simulink model "D_20210914_Modell_Inbetriebnahme_BreakOutBox_Jetson"  (R2021a)
settings: Solver=ode1  StartTime=0.0  StopTime=500  FixedStep=Ts  RelTol=1e-3
PreLoadFcn:
  | pulsePeriod = 0.05;
  | 
  | Ts = 0.001;
  | 
  | FPGA_Frequency = 75000000;
  | 
  | ts_IO691 = 5e-3;
PostLoadFcn:
  | ewolfSetUp
InitFcn:
  | pulsePeriod = 0.05;
  | 
  | Ts = 0.001;
  | 
  | FPGA_Frequency = 75000000;
  | 
  | ts_IO691 = 5e-3;
StopFcn:
  | Simulink.sdi.clearPreferences;
  | if isfile(['sdi_view_',bdroot,'.mldatx'])
  | Simulink.sdi.view;
  | pause(3);
  | Simulink.sdi.loadView(['sdi_view_',bdroot,]);
  | end
values from neighbouring files (symbols this model uses):
  max_ac = 2    [ewolfSetUp.m]
  max_steer = 0.26    [ewolfSetUp.m]
  min_ac = -3    [ewolfSetUp.m]
  min_steer = -0.26    [ewolfSetUp.m]
  PredictionHorizon = 30    [ewolfSetUp.m]
undefined symbols (not defined in the file or in its folder): canChannel, DiscIntNeverNeededParam, Ended, HS, IO291, IO397, Single
libraries: lllalib x255, canmsglib x143, simulink x33, speedgoatlib_IO191 x5, speedgoatlib_IO291 x5, speedgoatlib_IO691 x3, slrealtimeiplib x2, simulink_extras x1, speedgoatlib_fpga_dio x1, speedgoatlib_fpga_quadrature x1, speedgoatlib_fpga x1, canlib x1
(part 7 of 7)

== system D_20210914_Modell_Inbetriebnahme_BreakOutBox_Jetson/IO691/CAN Read Loop - Port 3/Enabled Subsystem/extract radar data from CAN msg stream/Subsystem100/Subsystem9 ==
  reset : Inport
  data : Inport  Port=2
  saveBool : Inport  Port=3
  Mux : Mux  Inputs=10
  saveData{,1..9} (10 alike) : lllalib/saveData  SystemSampleTime=-1  VariantActivationTime=update diagram  Latency=0  AutoFrameSizeCalculation=off
  out : Outport
  nextSave : Outport  Port=2
  wires:
  saveData3/2 -> Mux/4
  saveData8/1 -> saveData9/2
  saveData7/1 -> saveData8/2
  reset/1 -> saveData/1, saveData1/1, saveData2/1, saveData3/1, saveData4/1, saveData5/1, saveData6/1, saveData8/1, saveData9/1, saveData7/1
  saveData3/1 -> saveData4/2
  saveData4/1 -> saveData5/2
  saveData2/2 -> Mux/3
  Mux/1 -> out/1
  saveData6/2 -> Mux/7
  saveData9/1 -> nextSave/1
  saveData4/2 -> Mux/5
  saveData5/1 -> saveData6/2
  saveData/2 -> Mux/1
  saveData8/2 -> Mux/9
  data/1 -> saveData/2
  saveData7/2 -> Mux/8
  saveData/1 -> saveData1/2
  saveData9/2 -> Mux/10
  saveData6/1 -> saveData7/2
  saveData2/1 -> saveData3/2
  saveData5/2 -> Mux/6
  saveData1/1 -> saveData2/2
  saveData1/2 -> Mux/2
  saveBool/1 -> saveData/3, saveData1/3, saveData2/3, saveData3/3, saveData4/3, saveData5/3, saveData6/3, saveData7/3, saveData8/3, saveData9/3

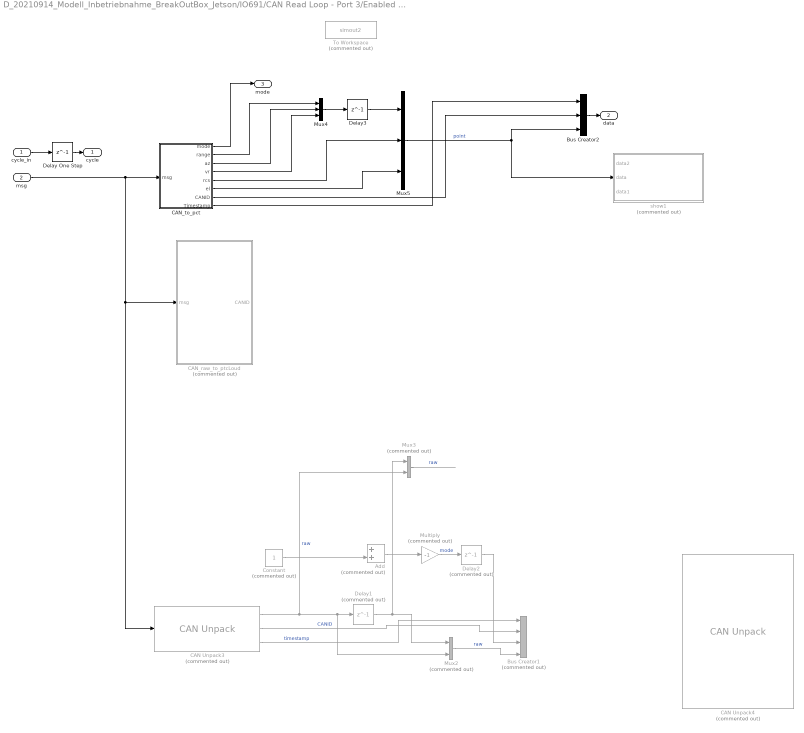
== system D_20210914_Modell_Inbetriebnahme_BreakOutBox_Jetson/IO691/CAN Read Loop - Port 3/Enabled Subsystem/extract radar data from CAN msg stream/extract point from CAN msg/extract radar_CAN_data (each cycle) ==
  cycle_in : Inport
  msg : Inport  Port=2
  Add : Sum  Commented=on
  Bus Creator1 : BusCreator  Commented=on  Inputs=4
  Bus Creator2 : BusCreator  Inputs=3
  CAN Unpack3 : canmsglib/CAN Unpack  Commented=on  MsgList=(none)  MsgName=CAN Msg  MsgIDType=Standard (11-bit identifier)  MsgIdentifier=-1  MsgLength=8  SignalInfo={}  IDPort=on  TimestampPort=on  ErrorPort=off  RemotePort=off  LengthPort=off  StatusPort=off  ApplyMinMax=off
      settings: SourceProductBaseCode=ME,XP,VN  DataFormat=raw data
  CAN Unpack4 : canmsglib/CAN Unpack  Commented=on  MsgList=(none)  MsgName=CAN Msg  MsgIDType=Standard (11-bit identifier)  MsgIdentifier=-1  MsgLength=8  SignalInfo={ 'Mode', '0', '1', 'LE', 'unsigned', 'Multiplexor', '0', '1', '0', '-Inf', 'Inf'; 'Range', '1', '13', 'LE', 'unsigned', 'Multiplexed', '0', '0.04', '0', '-Inf', 'Inf'; 'int1', '14', '8', 'LE', 'unsigned', 'Multiplexed', '0', '1', '0', '-Inf', 'Inf'; 'az', '22', '10', 'LE', 'unsigned', 'Multiplexed', '0', '1', '0', '-Inf', 'Inf'; 'int2', '32', '7', 'LE', 'unsigned', 'Multiplexed', '0', '1', '0', '-Inf', 'Inf'; 'vr', '39', '12', 'LE', 'unsigned', 'Multiplexed', '0', '0.04', '2992', '-44.12', '119.68'; 'int3', '51', '7', 'LE', 'unsigned', 'Multiplexed', '0', '1', '0', '-Inf', 'Inf'; 'int4', '58', '6', 'LE', 'unsigned', 'Multiplexed', '0', '1', '0', '-Inf', 'Inf'; 'rcs', '1', '8', 'LE', 'unsigned', 'Multiplexed', '1', '0.2', '75', '-15', '36'; 'int5', '9', '8', 'LE', 'unsigned', 'Multiplexed', '1', '1', '0', '-Inf', 'Inf'; 'int6', '17', '8', 'LE', 'unsigned', 'Multiplexed', '1', '1', '0', '-Inf', 'Inf'; 'int7', '25', '7', 'LE', 'unsigned', 'Multiplexed', '1', '1', '0', '-Inf', 'Inf'; 'resev', '32', '5', 'LE', 'unsigned', 'Multiplexed', '1', '1', '0', '-Inf', 'Inf'; 'elev', '37', '10', 'LE', 'unsigned', 'Multiplexed', '1', '0.04', '511', '-20.44', '20.48'; 'resev', '47', '17', 'LE', 'unsigned', 'Multiplexed', '1', '1', '0', '-Inf', 'Inf' }  IDPort=on  TimestampPort=on  ErrorPort=off  RemotePort=off  LengthPort=off  StatusPort=off  ApplyMinMax=off
      settings: SourceProductBaseCode=ME,XP,VN
  CAN_raw_to_ptcLoud : MATLAB Function  Commented=on  TreatAsAtomicUnit=on
  CAN_to_pct : MATLAB Function  TreatAsAtomicUnit=on
  Constant : Constant  Commented=on
  Delay One Step : Delay  DelayLength=1
  Delay1 : Delay  Commented=on  DelayLength=1  InitialCondition=0
  Delay2 : Delay  Commented=on  DelayLength=1  InitialCondition=0
  Delay3 : Delay  DelayLength=1  InitialCondition=0
  Multiply : Gain  Commented=on  Gain=-1
  Mux2 : Mux  Commented=on  Inputs=2
  Mux3 : Mux  Commented=on  Inputs=2
  Mux4 : Mux  Inputs=3
  Mux5 : Mux  Inputs=3
  To Workspace : ToWorkspace  Commented=on  VariableName=simout2  SaveFormat=Timeseries  SampleTime=-1
  show1 : MATLAB Function  Commented=on  TreatAsAtomicUnit=on
  cycle : Outport
  data : Outport  Port=2
  mode : Outport  Port=3
  wires:
  Delay One Step/1 -> cycle/1
  cycle_in/1 -> Delay One Step/1
  CAN_to_pct/8(Timestamp) -> Bus Creator2/1
  CAN_to_pct/7(CANID) -> Bus Creator2/2
  CAN_to_pct/6(el) -> Mux5/3
  CAN_to_pct/5(rcs) -> Mux5/2
  CAN_to_pct/4(vr) -> Mux4/3
  CAN_to_pct/3(az) -> Mux4/2
  CAN_to_pct/2(range) -> Mux4/1
  CAN_to_pct/1(mode) -> mode/1
  Bus Creator2/1 -> data/1
  Delay3/1 -> Mux5/1
  Mux5/1 -> show1/2(data), Bus Creator2/3  "point"
  Mux4/1 -> Delay3/1
  Mux3/1 -> ?  "raw"
  Delay2/1 -> Bus Creator1/3
  Multiply/1 -> Delay2/1  "mode"
  Add/1 -> Multiply/1
  Constant/1 -> Add/2
  CAN Unpack3/2 -> Bus Creator1/2  "CANID"
  CAN Unpack3/3 -> Bus Creator1/1  "timestamp"
  Mux2/1 -> Bus Creator1/4  "raw"
  Delay1/1 -> Mux2/1, Mux3/1
  CAN Unpack3/1 -> Delay1/1, Mux2/2, Mux3/2  "raw"
  msg/1 -> CAN_to_pct/1(msg), CAN_raw_to_ptcLoud/1(msg), CAN Unpack3/1

== system D_20210914_Modell_Inbetriebnahme_BreakOutBox_Jetson/IO691/CAN Read Loop - Port 3/Enabled Subsystem/extract radar data from CAN msg stream/save 55/Subsystem ==
  reset : Inport
  data : Inport  Port=2
  saveBool : Inport  Port=3
  Mux : Mux  Inputs=10
  saveData{,1..9} (10 alike) : lllalib/saveData  SystemSampleTime=-1  VariantActivationTime=update diagram  Latency=0  AutoFrameSizeCalculation=off
  out : Outport
  nextSave : Outport  Port=2
  wires:
  saveData3/2 -> Mux/4
  saveData8/1 -> saveData9/2
  saveData7/1 -> saveData8/2
  reset/1 -> saveData/1, saveData1/1, saveData2/1, saveData3/1, saveData4/1, saveData5/1, saveData6/1, saveData8/1, saveData9/1, saveData7/1
  saveData3/1 -> saveData4/2
  saveData4/1 -> saveData5/2
  saveData2/2 -> Mux/3
  Mux/1 -> out/1
  saveData6/2 -> Mux/7
  saveData9/1 -> nextSave/1
  saveData4/2 -> Mux/5
  saveData5/1 -> saveData6/2
  saveData/2 -> Mux/1
  saveData8/2 -> Mux/9
  data/1 -> saveData/2
  saveData7/2 -> Mux/8
  saveData/1 -> saveData1/2
  saveData9/2 -> Mux/10
  saveData6/1 -> saveData7/2
  saveData2/1 -> saveData3/2
  saveData5/2 -> Mux/6
  saveData1/1 -> saveData2/2
  saveData1/2 -> Mux/2
  saveBool/1 -> saveData/3, saveData1/3, saveData2/3, saveData3/3, saveData4/3, saveData5/3, saveData6/3, saveData7/3, saveData8/3, saveData9/3

== system D_20210914_Modell_Inbetriebnahme_BreakOutBox_Jetson/IO691/CAN Read Loop - Port 3/Enabled Subsystem/extract radar data from CAN msg stream/save 55/Subsystem1 ==
  reset : Inport
  data : Inport  Port=2
  saveBool : Inport  Port=3
  Mux : Mux  Inputs=10
  saveData{,1..9} (10 alike) : lllalib/saveData  SystemSampleTime=-1  VariantActivationTime=update diagram  Latency=0  AutoFrameSizeCalculation=off
  out : Outport
  nextSave : Outport  Port=2
  wires:
  saveData3/2 -> Mux/4
  saveData8/1 -> saveData9/2
  saveData7/1 -> saveData8/2
  reset/1 -> saveData/1, saveData1/1, saveData2/1, saveData3/1, saveData4/1, saveData5/1, saveData6/1, saveData8/1, saveData9/1, saveData7/1
  saveData3/1 -> saveData4/2
  saveData4/1 -> saveData5/2
  saveData2/2 -> Mux/3
  Mux/1 -> out/1
  saveData6/2 -> Mux/7
  saveData9/1 -> nextSave/1
  saveData4/2 -> Mux/5
  saveData5/1 -> saveData6/2
  saveData/2 -> Mux/1
  saveData8/2 -> Mux/9
  data/1 -> saveData/2
  saveData7/2 -> Mux/8
  saveData/1 -> saveData1/2
  saveData9/2 -> Mux/10
  saveData6/1 -> saveData7/2
  saveData2/1 -> saveData3/2
  saveData5/2 -> Mux/6
  saveData1/1 -> saveData2/2
  saveData1/2 -> Mux/2
  saveBool/1 -> saveData/3, saveData1/3, saveData2/3, saveData3/3, saveData4/3, saveData5/3, saveData6/3, saveData7/3, saveData8/3, saveData9/3

== system D_20210914_Modell_Inbetriebnahme_BreakOutBox_Jetson/IO691/CAN Read Loop - Port 3/Enabled Subsystem/extract radar data from CAN msg stream/save 55/Subsystem2 ==
  reset : Inport
  data : Inport  Port=2
  saveBool : Inport  Port=3
  Mux : Mux  Inputs=10
  saveData{,1..9} (10 alike) : lllalib/saveData  SystemSampleTime=-1  VariantActivationTime=update diagram  Latency=0  AutoFrameSizeCalculation=off
  out : Outport
  nextSave : Outport  Port=2
  wires:
  saveData3/2 -> Mux/4
  saveData8/1 -> saveData9/2
  saveData7/1 -> saveData8/2
  reset/1 -> saveData/1, saveData1/1, saveData2/1, saveData3/1, saveData4/1, saveData5/1, saveData6/1, saveData8/1, saveData9/1, saveData7/1
  saveData3/1 -> saveData4/2
  saveData4/1 -> saveData5/2
  saveData2/2 -> Mux/3
  Mux/1 -> out/1
  saveData6/2 -> Mux/7
  saveData9/1 -> nextSave/1
  saveData4/2 -> Mux/5
  saveData5/1 -> saveData6/2
  saveData/2 -> Mux/1
  saveData8/2 -> Mux/9
  data/1 -> saveData/2
  saveData7/2 -> Mux/8
  saveData/1 -> saveData1/2
  saveData9/2 -> Mux/10
  saveData6/1 -> saveData7/2
  saveData2/1 -> saveData3/2
  saveData5/2 -> Mux/6
  saveData1/1 -> saveData2/2
  saveData1/2 -> Mux/2
  saveBool/1 -> saveData/3, saveData1/3, saveData2/3, saveData3/3, saveData4/3, saveData5/3, saveData6/3, saveData7/3, saveData8/3, saveData9/3

== system D_20210914_Modell_Inbetriebnahme_BreakOutBox_Jetson/IO691/CAN Read Loop - Port 3/Enabled Subsystem/extract radar data from CAN msg stream/save 55/Subsystem3 ==
  reset : Inport
  data : Inport  Port=2
  saveBool : Inport  Port=3
  Mux : Mux  Inputs=10
  saveData{,1..9} (10 alike) : lllalib/saveData  SystemSampleTime=-1  VariantActivationTime=update diagram  Latency=0  AutoFrameSizeCalculation=off
  out : Outport
  nextSave : Outport  Port=2
  wires:
  saveBool/1 -> saveData9/3, saveData8/3, saveData7/3, saveData6/3, saveData5/3, saveData4/3, saveData3/3, saveData2/3, saveData1/3, saveData/3
  saveData1/2 -> Mux/2
  saveData1/1 -> saveData2/2
  saveData5/2 -> Mux/6
  saveData2/1 -> saveData3/2
  saveData6/1 -> saveData7/2
  saveData9/2 -> Mux/10
  saveData/1 -> saveData1/2
  saveData7/2 -> Mux/8
  data/1 -> saveData/2
  saveData8/2 -> Mux/9
  saveData/2 -> Mux/1
  saveData5/1 -> saveData6/2
  saveData4/2 -> Mux/5
  saveData9/1 -> nextSave/1
  saveData6/2 -> Mux/7
  Mux/1 -> out/1
  saveData2/2 -> Mux/3
  saveData4/1 -> saveData5/2
  saveData3/1 -> saveData4/2
  reset/1 -> saveData7/1, saveData9/1, saveData8/1, saveData6/1, saveData5/1, saveData4/1, saveData3/1, saveData2/1, saveData1/1, saveData/1
  saveData7/1 -> saveData8/2
  saveData8/1 -> saveData9/2
  saveData3/2 -> Mux/4

== system D_20210914_Modell_Inbetriebnahme_BreakOutBox_Jetson/IO691/CAN Read Loop - Port 3/Enabled Subsystem/extract radar data from CAN msg stream/save 55/Subsystem4 ==
  reset : Inport
  data : Inport  Port=2
  saveBool : Inport  Port=3
  Mux : Mux  Inputs=10
  saveData{,1..9} (10 alike) : lllalib/saveData  SystemSampleTime=-1  VariantActivationTime=update diagram  Latency=0  AutoFrameSizeCalculation=off
  out : Outport
  nextSave : Outport  Port=2
  wires:
  saveData3/2 -> Mux/4
  saveData8/1 -> saveData9/2
  saveData7/1 -> saveData8/2
  reset/1 -> saveData/1, saveData1/1, saveData2/1, saveData3/1, saveData4/1, saveData5/1, saveData6/1, saveData8/1, saveData9/1, saveData7/1
  saveData3/1 -> saveData4/2
  saveData4/1 -> saveData5/2
  saveData2/2 -> Mux/3
  Mux/1 -> out/1
  saveData6/2 -> Mux/7
  saveData9/1 -> nextSave/1
  saveData4/2 -> Mux/5
  saveData5/1 -> saveData6/2
  saveData/2 -> Mux/1
  saveData8/2 -> Mux/9
  data/1 -> saveData/2
  saveData7/2 -> Mux/8
  saveData/1 -> saveData1/2
  saveData9/2 -> Mux/10
  saveData6/1 -> saveData7/2
  saveData2/1 -> saveData3/2
  saveData5/2 -> Mux/6
  saveData1/1 -> saveData2/2
  saveData1/2 -> Mux/2
  saveBool/1 -> saveData/3, saveData1/3, saveData2/3, saveData3/3, saveData4/3, saveData5/3, saveData6/3, saveData7/3, saveData8/3, saveData9/3

== system D_20210914_Modell_Inbetriebnahme_BreakOutBox_Jetson/IO691/CAN Read Loop - Port 3/Enabled Subsystem/extract radar data from CAN msg stream/save 55/Subsystem5 ==
  reset : Inport
  data : Inport  Port=2
  saveBool : Inport  Port=3
  Mux : Mux  Inputs=5
  saveData{,1..4} (5 alike) : lllalib/saveData  SystemSampleTime=-1  VariantActivationTime=update diagram  Latency=0  AutoFrameSizeCalculation=off
  out : Outport
  wires:
  saveBool/1 -> saveData4/3, saveData3/3, saveData2/3, saveData1/3, saveData/3
  saveData1/2 -> Mux/2
  saveData1/1 -> saveData2/2
  saveData2/1 -> saveData3/2
  saveData/1 -> saveData1/2
  data/1 -> saveData/2
  saveData/2 -> Mux/1
  saveData4/2 -> Mux/5
  Mux/1 -> out/1
  saveData2/2 -> Mux/3
  saveData3/1 -> saveData4/2
  reset/1 -> saveData4/1, saveData3/1, saveData2/1, saveData1/1, saveData/1
  saveData3/2 -> Mux/4

== matlab function D_20210914_Modell_Inbetriebnahme_BreakOutBox_Jetson/Nvidia_Jetson/LaneFollowingAndControl/Estimate Lane Center1/MATLAB Function1 ==
  data: lanes input
  events: fcnLeftAndRight output FUNCTION_CALL_EVENT; fcnLeftOnly output FUNCTION_CALL_EVENT; fcnRightOnly output FUNCTION_CALL_EVENT; fcnNone output FUNCTION_CALL_EVENT
function fcn(lanes)

leftStrength  = lanes.Left.Strength;
rightStrength = lanes.Right.Strength;

if (leftStrength > 0) && (rightStrength > 0)
   fcnLeftAndRight();
   
elseif leftStrength > 0
    fcnLeftOnly();
    
elseif rightStrength > 0
    fcnRightOnly();
    
else
    fcnNone();
end

== matlab function D_20210914_Modell_Inbetriebnahme_BreakOutBox_Jetson/IO691/CAN Read Loop - Port 3/Enabled Subsystem/extract radar data from CAN msg stream/extract point from CAN msg/extract radar_CAN_data (each cycle)/CAN_raw_to_ptcLoud ==
  data: msg input uint8 size=8; CANID output uint8
function CANID = CAN_raw_to_ptcLoud(msg)
% ,range,az,vr,rcs,el,
% mode = -1;
CANID = 0;
Timestamp = 0;
% CANID = msg.ID;
% Timestamp = msg.Timestamp;

data = msg.Data;
bb = dec2bin([data]);
rBB = reshape(flip(bb'),1,[]);

disp(rBB(1));

% mode = rBB(1);
% % Mode = 0
% range = (bin2dec(flip(rBB(2:14))))*0.04; % range: res = 0.04 m, Offset = 0
% az = (bin2dec(flip(rBB(23:32)))-511)*0.04; % azimuth: res = 0.16 °, Offset = 511
% vr = (bin2dec(flip(rBB(40:51)))-2992)*0.04; % vr: res = 0.04 m/s, Offset = 2992
% 
% 
% % Mode = 1
% rcs = (bin2dec(flip(rBB(2:9)))-75)*0.2; % rcs: res = 0.2 dB, Offset = 75
% el = (bin2dec(flip(rBB(38:47)))-511)*0.16; % range: res = 0.16 °, Offset = 511

== matlab function D_20210914_Modell_Inbetriebnahme_BreakOutBox_Jetson/IO691/CAN Read Loop - Port 3/Enabled Subsystem/extract radar data from CAN msg stream/extract point from CAN msg/extract radar_CAN_data (each cycle)/CAN_to_pct ==
  data: msg input; mode output; range output; az output; vr output; rcs output; el output; CANID output; Timestamp output
function [mode,range,az,vr,rcs,el,CANID,Timestamp] = fcn(msg)
% Lukas Lang, 04.04.2022
% Matlab/Simulink function to extract radar data from smartmicro's UMRR
% radar msg:
% - input: msg = CAN msg (struct with CAN_ID, tmiestamp, length, data, etc
%           ....
% - output: mode,range,az,vr,rcs,el,CANID,Timestamp = extracted radar data
% ( see Customer_interface_V02.pdf)
%   return mode == 0 if CAN ID not between double(1025:1279) /
%   hex(0x401:0x4FF) || data length ~= 8 Byte

CANID = 0;
Timestamp = 0;
mode = 0;
range = -1;
az = 0;
vr = 0;
rcs = 0;
el = 0;
CANID = 0;
Timestamp = 0;
CANID = double(msg.ID);

if isempty(find(1025:1279==CANID))  % return mode == -1 if CAN msg no smartmicro UMRR radar msg!!
    return;
end


Timestamp = double(msg.Timestamp);

data = msg.Data;
bb = dec2bin([data]);
rBB = reshape(flip(bb'),1,[]);

if length(rBB)~=64
    return;
end
% disp('-----------------------')
% disp(rBB);
% disp('-----------------------')
mode = bin2dec(rBB(1));

range = (bin2dec(flip(rBB(2:14))))*0.04; % range: res = 0.04 m, Offset = 0
az = (bin2dec(flip(rBB(23:32)))-511)*0.16; % azimuth: res = 0.16 °, Offset = 511
vr = (bin2dec(flip(rBB(40:51)))-2992)*0.04; % vr: res = 0.04 m/s, Offset = 2992


% Mode = 1
rcs = (bin2dec(flip(rBB(2:9)))-75)*0.2; % rcs: res = 0.2 dB, Offset = 75
el = (bin2dec(flip(rBB(38:47)))-511)*0.04; % range: res = 0.16 °, Offset = 511

== stateflow chart D_20210914_Modell_Inbetriebnahme_BreakOutBox_Jetson/Bremspedal Steuerung/QAD Steuerung1/QAD1/State Transition Table ==
  state state_0_0
  state state_1_0
  state state_1_1
  state state_0_1
  (default) -> state_0_0 [order 1] : [Hall_A==0 & Hall_B==0]
  state_0_0 -> (junction 72) [order 3] : [Hall_A==0 & Hall_B==0]
      | {count_enable=0; count_dir=2}
  (junction 72) -> state_0_0
  (junction 76) -> state_0_0
  state_0_0 -> (junction 69) [order 2] : [Hall_A==0 & Hall_B==1]
      | {count_enable=1; count_dir=0}
  (junction 126) -> (junction 76)
  (junction 69) -> (junction 129)
  state_0_0 -> (junction 134) [order 4] : [Hall_A==1 & Hall_B==1]
      | {count_enable=0; count_dir=2}
  (junction 134) -> (junction 132)
  state_0_0 -> state_1_0 [order 1] : [Hall_A==1 & Hall_B==0]
      | {count_enable=1; count_dir=1}
  state_1_0 -> state_0_0 [order 2] : [Hall_A==0 & Hall_B==0]
      | {count_enable=1; count_dir=0}
  (default) -> state_1_0 [order 2] : [Hall_A==1 & Hall_B==0]
  state_1_0 -> (junction 43) [order 3] : [Hall_A==1 & Hall_B==0]
      | {count_enable=0; count_dir=2}
  (junction 43) -> state_1_0
  (junction 121) -> state_1_0
  (junction 123) -> (junction 121)
  state_1_0 -> (junction 129) [order 4] : [Hall_A==0 & Hall_B==1]
      | {count_enable=0; count_dir=2}
  (junction 129) -> (junction 67)
  state_1_0 -> state_1_1 [order 1] : [Hall_A==1 & Hall_B==1]
      | {count_enable=1; count_dir=1}
  state_1_1 -> state_1_0 [order 2] : [Hall_A==1 & Hall_B==0]
      | {count_enable=1; count_dir=0}
  (default) -> state_1_1 [order 3] : [Hall_A==1 & Hall_B==1]
  state_1_1 -> (junction 47) [order 3] : [Hall_A==1 & Hall_B==1]
      | {count_enable=0; count_dir=2}
  (junction 47) -> state_1_1
  state_1_1 -> (junction 126) [order 4] : [Hall_A==0 & Hall_B==0]
      | {count_enable=0; count_dir=2}
  (junction 78) -> (junction 126)
  (junction 132) -> state_1_1
  state_1_1 -> state_0_1 [order 1] : [Hall_A==0 & Hall_B==1]
      | {count_enable=1; count_dir=1}
  state_0_1 -> state_1_1 [order 2] : [Hall_A==1 & Hall_B==1]
      | {count_enable=1; count_dir=0}
  (default) -> state_0_1 [order 4]
  state_0_1 -> (junction 50) [order 3] : [Hall_A==0 & Hall_B==1]
      | {count_enable=0; count_dir=2}
  (junction 50) -> state_0_1
  state_0_1 -> (junction 78) [order 1] : [Hall_A==0 & Hall_B==0]
      | {count_enable=1; count_dir=1}
  state_0_1 -> (junction 123) [order 4] : [Hall_A==1 & Hall_B==0]
      | {count_enable=0; count_dir=2}
  (junction 67) -> state_0_1
  data: Hall_A input; Hall_B input; count_enable output; count_dir output

== matlab function D_20210914_Modell_Inbetriebnahme_BreakOutBox_Jetson/IO691/CAN Read Loop - Port 3/Enabled Subsystem/extract radar data from CAN msg stream/extract point from CAN msg/extract radar_CAN_data (each cycle)/show1 ==
  data: data2 input; data input; data1 input
function unpackRadarCAN(data2, data, data1)

if data1 == 1
    disp('last. ####')
    disp(data2)
    disp(data)
    disp('last. ####')
end

== matlab function D_20210914_Modell_Inbetriebnahme_BreakOutBox_Jetson/IO691/CAN Read Loop - Port 3/Enabled Subsystem/extract radar data from CAN msg stream/extract point from CAN msg/if_header_msg ==
  data: isHeader output; msg input; cycl input; numObj input
function isHeader   = unpackRadarCAN(msg,cycl, numObj)

isHeader = 1;
if msg.ID~=1024
%     disp('next. ####')
%     disp(msg.ID)
    isHeader = 0;
end

== matlab function D_20210914_Modell_Inbetriebnahme_BreakOutBox_Jetson/Nvidia_Jetson/MATLAB Function ==
  data: u input; y output
function y = fcn(u)
% u input message uint8
% y output lane parameter
y = zeros(1,6);
u1 = u(1:8);
u2 = u(9:16);
u3 = u(17:24);
u4 = u(25:32);
u5 = u(33:40);
u6 = u(41:48);

y(1) = typecast( uint8(u1) , 'double');
y(2) = typecast( uint8(u2) , 'double');
y(3) = typecast( uint8(u3) , 'double');
y(4) = typecast( uint8(u4) , 'double');
y(5) = typecast( uint8(u5) , 'double');
y(6) = typecast( uint8(u6) , 'double');
